simulink model "test"  (R2023b)
settings: Solver=VariableStepAuto  StartTime=0.0  StopTime=10.0  RelTol=1e-3
settings Model: Creator=arnaud  LastModifiedBy=arnaud

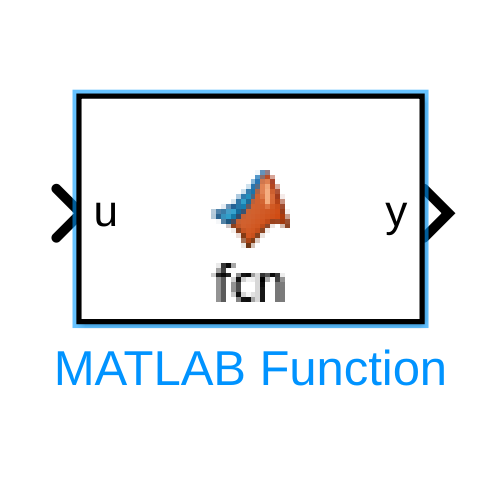
[thumbnail: Simulink's stored preview of the top-level diagram]
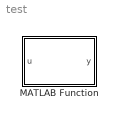
== system test ==
  MATLAB Function : MATLAB Function  TreatAsAtomicUnit=on

== matlab function test/MATLAB Function ==
  data: u input; y output
function y = fcn(u)

y = directions+u;

end
